simulink model "path_tracker_demo"  (R2019b)
settings: Solver=FixedStepDiscrete  StartTime=0.0  StopTime=40  FixedStep=0.01  RelTol=1e-3  EnableMultiTasking=on
undefined symbols (not defined in the file or in its folder): DiscIntNeverNeededParam, path_data_D
libraries: simulink x3
Description:
  | Counter Implemented in a C++ S-function
settings Model: ExtModeTrigMode=oneshot  ExtModeArmWhenConnect=off  ExtModeAutoUpdateStatusClock=off  Creator=The MathWorks, Inc.  LastModifiedBy=chr
settings DataIOCC: SaveFormat=Array
settings OptimizationCC: BlockReduction=off  BooleanDataType=off  ExpressionDepthLimit=2147483647  InitFltsAndDblsToZero=on  LifeSpan=inf
settings DebuggingCC: SaveWithParameterizedLinksMsg=none  SignalResolutionControl=TryResolveAllWithWarning  MultiTaskDSMMsg=warning  MultiTaskCondExecSysMsg=none  FcnCallInpInsideContextMsg=warning  StateNameClashWarn=warning  SFUnexpectedBacktrackingDiag=warning  SFNoUnconditionalDefaultTransitionDiag=warning  SFExecutionAtInitializationDiag=none  ArithmeticOperatorsInVariantConditions=warning
settings HardwareCC: ProdBitPerPointer=32  ProdBitPerSizeT=32  ProdBitPerPtrDiffT=32  ProdLargestAtomicFloat=None  ProdIntDivRoundTo=Undefined  ProdEndianess=Unspecified  ProdWordSize=32  ProdHWDeviceType=32-bit Generic
settings ModelReferenceCC: PropagateSignalLabelsOutOfModel=off
settings SFSimCC: SimUseLocalCustomCode=off  CustomCodeUndefinedFunction=UseInterfaceOnly
settings RTWCC: Description=Generic Real-Time Target  RetainRTWFile=on  RTWUseLocalCustomCode=off
settings CodeAppCC: StateflowObjectComments=on
settings GRTTargetCC: TargetFcnLib=ansi_tfl_tmw.mat  TargetLangStandard=C89/C90 (ANSI)  GeneratePreprocessorConditionals=Disable all  CombineOutputUpdateFcns=off  GRTInterface=on
settings ConfigComp: CovMetricSettings=dw  CovHtmlReporting=on  CovSaveCumulativeToWorkspaceVar=on  CovSaveSingleToWorkspaceVar=on  CovExternalEMLEnable=off

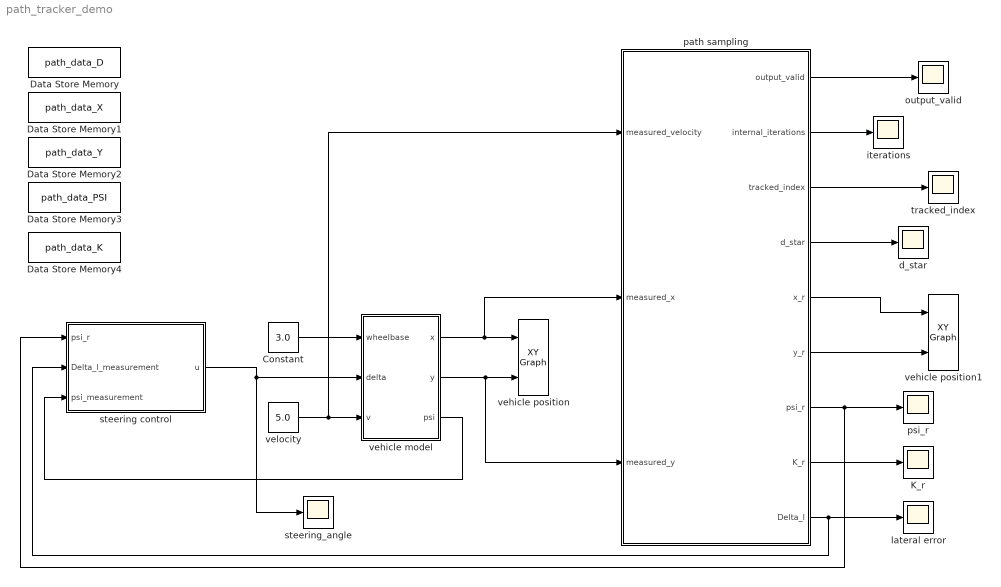
== system path_tracker_demo ==
  Constant : Constant  Value=3.0
  Data Store Memory : DataStoreMemory  DataStoreName=path_data_D  ReadBeforeWriteMsg=warning  WriteAfterWriteMsg=warning  WriteAfterReadMsg=warning  InitialValue=path_data.D  ShowAdditionalParam=off
  Data Store Memory1 : DataStoreMemory  DataStoreName=path_data_X  ReadBeforeWriteMsg=warning  WriteAfterWriteMsg=warning  WriteAfterReadMsg=warning  InitialValue=path_data.X  ShowAdditionalParam=off
  Data Store Memory2 : DataStoreMemory  DataStoreName=path_data_Y  ReadBeforeWriteMsg=warning  WriteAfterWriteMsg=warning  WriteAfterReadMsg=warning  InitialValue=path_data.Y  ShowAdditionalParam=off
  Data Store Memory3 : DataStoreMemory  DataStoreName=path_data_PSI  ReadBeforeWriteMsg=warning  WriteAfterWriteMsg=warning  WriteAfterReadMsg=warning  InitialValue=path_data.PSI  ShowAdditionalParam=off
  Data Store Memory4 : DataStoreMemory  DataStoreName=path_data_K  ReadBeforeWriteMsg=warning  WriteAfterWriteMsg=warning  WriteAfterReadMsg=warning  InitialValue=path_data.K  ShowAdditionalParam=off
  K_r : Scope
  d_star : Scope
  iterations : Scope
  lateral error : Scope
  output_valid : Scope
  path sampling : Subsystem
  psi_r : Scope
  steering control : Subsystem
  steering_angle : Scope
  tracked_index : Scope
  vehicle position : simulink/Sinks/XY Graph  xmin=-40  xmax=40  ymin=-40  ymax=40  st=-1
  vehicle position1 : simulink/Sinks/XY Graph  xmin=-40  xmax=40  ymin=-40  ymax=40  st=-1
  vehicle model : Subsystem
  velocity : Constant  Value=5.0
  wires:
  path sampling/1(output_valid) -> output_valid/1
  path sampling/2(internal_iterations) -> iterations/1
  path sampling/7(psi_r) -> steering control/1(psi_r), psi_r/1
  path sampling/8(K_r) -> K_r/1
  path sampling/3(tracked_index) -> tracked_index/1
  Constant/1 -> vehicle model/1(wheelbase)
  velocity/1 -> path sampling/1(measured_velocity), vehicle model/3(v)
  vehicle model/1(x) -> vehicle position/1, path sampling/2(measured_x)
  vehicle model/2(y) -> vehicle position/2, path sampling/3(measured_y)
  path sampling/5(x_r) -> vehicle position1/1
  path sampling/6(y_r) -> vehicle position1/2
  path sampling/9(Delta_l) -> steering control/2(Delta_l_measurement), lateral error/1
  path sampling/4(d_star) -> d_star/1
  steering control/1(u) -> steering_angle/1, vehicle model/2(delta)
  vehicle model/3(psi) -> steering control/3(psi_measurement)

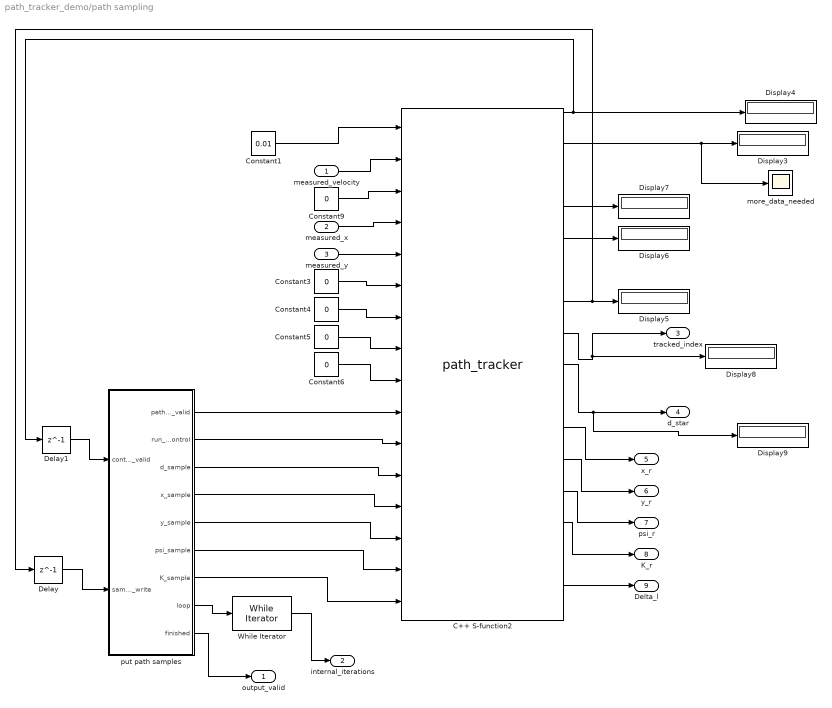
== system path_tracker_demo/path sampling ==
  measured_velocity : Inport
  measured_x : Inport  Port=2
  measured_y : Inport  Port=3
  C++ S-function2 : S-Function  FunctionName=path_tracker  Parameters=-1  SFunctionDeploymentMode=off  EnableBusSupport=off
      mask Display:
      | % copy and paste these commands into the field 'icon drawing commands' of the block mask:
      | % right-click on block -> 'Mask' -> 'Edit Mask' -> 'Mask Editor' -> 'Icons & Ports'
      | 
      | port_label('input', 1, 'Ts')
      | port_label('input', 2, 'velocity_')
      | port_label('input', 3, 'velocity_dot')
      | port_label('input', 4, 'x')
      | port_label('input', 5, 'y')
      | port_label('input', 6, 'x_dot')
      | port_label('input', 7, 'y_dot')
      | port_label('input', 8, 'Delta_u')
      | port_label('input', 9, 'Delta_u_dot')
      | port_label('input', 10, 'async_input_data_valid')
      | port_label('input', 11, 'input_sample_valid')
      | port_label('input', 12, 'd_sample')
      | port_label('input', 13, 'x_sample')
      | port_label('input', 14, 'y_sample')
      | port_label('input', 15, 'psi_sample')
      | port_label('input', 16, 'K_sample')
      | port_label('output', 1, 'output_valid')
      | port_label('output', 2, 'need_more_path_input_data')
      | port_label('output', 3, 'distance_at_the_end_of_horizon')
      | port_label('output', 4, 'distance_ahead')
      | port_label('output', 5, 'head_index')
      | port_label('output', 6, 'read_position')
      | port_label('output', 7, 'elements_free_to_write')
      | port_label('output', 8, 'tracked_index')
      | port_label('output', 9, 'd_star')
      | port_label('output', 10, 'v_star')
      | port_label('output', 11, 'x_r')
      | port_label('output', 12, 'y_r')
      | port_label('output', 13, 'psi_r')
      | port_label('output', 14, 'K_r')
      | port_label('output', 15, 'psi_r_dot')
      | port_label('output', 16, 'Delta_l')
      | port_label('output', 17, 'Delta_l_dot')
  Constant1 : Constant  Value=0.01
  Constant{3..6,9} (5 alike) : Constant  Value=0
  Delay : Delay  DelayLength=1  InitialCondition=0
  Delay1 : Delay  DelayLength=1  InitialCondition=0
  Display{3..9} (7 alike) : Display
  While Iterator : WhileIterator  MaxIters=1000  WhileBlockType=do-while  ShowIterationPort=on
  more_data_needed : Scope
  put path samples : Subsystem
  output_valid : Outport
  internal_iterations : Outport  Port=2
  tracked_index : Outport  Port=3
  d_star : Outport  Port=4
  x_r : Outport  Port=5
  y_r : Outport  Port=6
  psi_r : Outport  Port=7
  K_r : Outport  Port=8
  Delta_l : Outport  Port=9
  wires:
  C++ S-function2/5 -> Display6/1
  Constant4/1 -> C++ S-function2/7
  measured_y/1 -> C++ S-function2/5
  Constant6/1 -> C++ S-function2/9
  C++ S-function2/8 -> Display8/1, tracked_index/1
  Constant3/1 -> C++ S-function2/6
  measured_velocity/1 -> C++ S-function2/2
  Constant1/1 -> C++ S-function2/1
  C++ S-function2/2 -> more_data_needed/1, Display3/1
  C++ S-function2/9 -> Display9/1, d_star/1
  Constant5/1 -> C++ S-function2/8
  C++ S-function2/7 -> Display5/1, Delay/1
  Constant9/1 -> C++ S-function2/3
  C++ S-function2/1 -> Display4/1, Delay1/1
  measured_x/1 -> C++ S-function2/4
  C++ S-function2/4 -> Display7/1
  While Iterator/1 -> internal_iterations/1
  put path samples/1(path_sample_valid) -> C++ S-function2/10
  put path samples/2(run_control) -> C++ S-function2/11
  put path samples/3(d_sample) -> C++ S-function2/12
  put path samples/4(x_sample) -> C++ S-function2/13
  put path samples/5(y_sample) -> C++ S-function2/14
  put path samples/6(psi_sample) -> C++ S-function2/15
  put path samples/7(K_sample) -> C++ S-function2/16
  put path samples/8(loop) -> While Iterator/1
  put path samples/9(finished) -> output_valid/1
  Delay/1 -> put path samples/2(samples_free_to_write)
  Delay1/1 -> put path samples/1(control_output_valid)
  C++ S-function2/14 -> K_r/1
  C++ S-function2/13 -> psi_r/1
  C++ S-function2/12 -> y_r/1
  C++ S-function2/11 -> x_r/1
  C++ S-function2/16 -> Delta_l/1

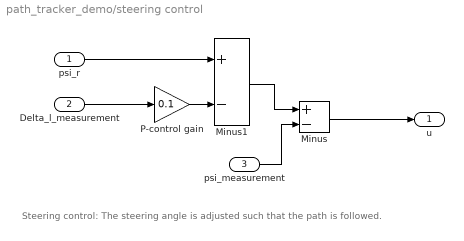
== system path_tracker_demo/steering control ==
  note: Steering control: The steering angle is adjusted such that the path is followed.
  psi_r : Inport
  Delta_l_measurement : Inport  Port=2
  psi_measurement : Inport  Port=3
  Minus : Sum  Inputs=+-
  Minus1 : Sum  Inputs=+-
  P-control gain : Gain  Gain=0.1
  u : Outport
  wires:
  psi_r/1 -> Minus1/1
  Minus/1 -> u/1
  P-control gain/1 -> Minus1/2
  psi_measurement/1 -> Minus/2
  Delta_l_measurement/1 -> P-control gain/1
  Minus1/1 -> Minus/1

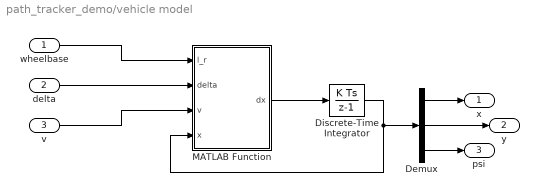
== system path_tracker_demo/vehicle model ==
  wheelbase : Inport
  delta : Inport  Port=2
  v : Inport  Port=3
  Demux : Demux  Outputs=[1;1;1]
  Discrete-Time Integrator : DiscreteIntegrator  InitialCondition=[0; 0; 0]  SampleTime=-1  ICPrevOutput=DiscIntNeverNeededParam  ICPrevScaledInput=DiscIntNeverNeededParam
  MATLAB Function : MATLAB Function  TreatAsAtomicUnit=on
  x : Outport
  y : Outport  Port=2
  psi : Outport  Port=3
  wires:
  Demux/1 -> x/1
  Demux/3 -> psi/1
  Demux/2 -> y/1
  wheelbase/1 -> MATLAB Function/1(l_r)
  delta/1 -> MATLAB Function/2(delta)
  MATLAB Function/1(dx) -> Discrete-Time Integrator/1
  v/1 -> MATLAB Function/3(v)
  Discrete-Time Integrator/1 -> Demux/1, MATLAB Function/4(x)

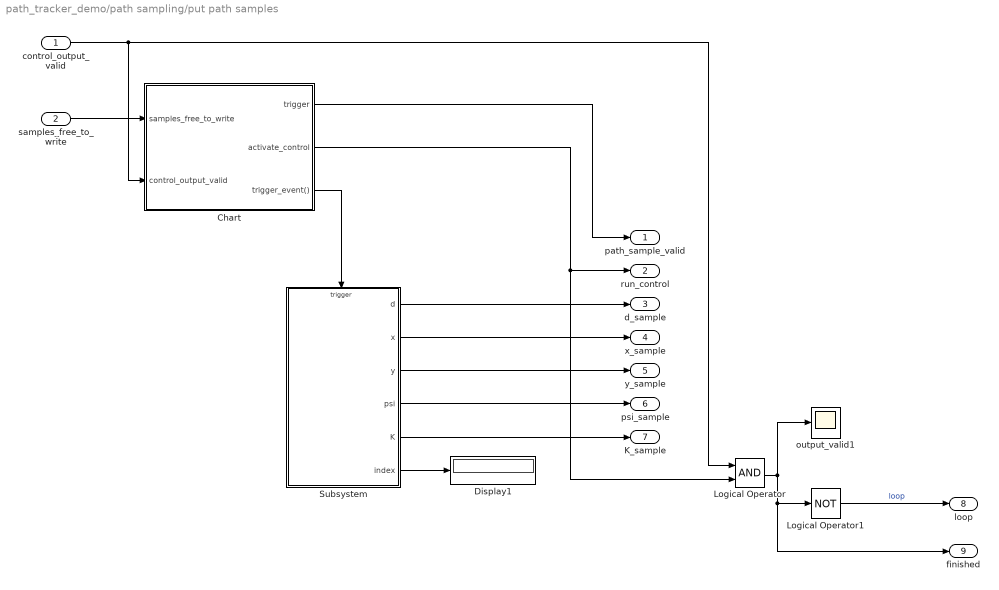
== system path_tracker_demo/path sampling/put path samples ==
  control_output_valid : Inport
  samples_free_to_write : Inport  Port=2
  Chart : Stateflow chart  BlockKeywords=__PRM__SERIALIZED__DATA__:Stateflow Chart,Stateflow Diagram  TreatAsAtomicUnit=on
  Display1 : Display
  Logical Operator : Logic  AllPortsSameDT=off  OutDataTypeStr=boolean
  Logical Operator1 : Logic  Operator=NOT  AllPortsSameDT=off  OutDataTypeStr=boolean
  Subsystem : Subsystem
  output_valid1 : Scope
  path_sample_valid : Outport
  run_control : Outport  Port=2
  d_sample : Outport  Port=3
  x_sample : Outport  Port=4
  y_sample : Outport  Port=5
  psi_sample : Outport  Port=6
  K_sample : Outport  Port=7
  loop : Outport  Port=8
  finished : Outport  Port=9
  wires:
  Logical Operator1/1 -> loop/1  "loop"
  Chart/1(trigger) -> path_sample_valid/1
  Subsystem/1(d) -> d_sample/1
  Subsystem/4(psi) -> psi_sample/1
  Subsystem/2(x) -> x_sample/1
  Subsystem/3(y) -> y_sample/1
  Subsystem/5(K) -> K_sample/1
  Logical Operator/1 -> finished/1, Logical Operator1/1, output_valid1/1
  control_output_valid/1 -> Chart/2(control_output_valid), Logical Operator/1
  Chart/2(activate_control) -> run_control/1, Logical Operator/2
  Subsystem/6(index) -> Display1/1
  Chart/3(trigger_event()) -> Subsystem/Trigger
  samples_free_to_write/1 -> Chart/1(samples_free_to_write)

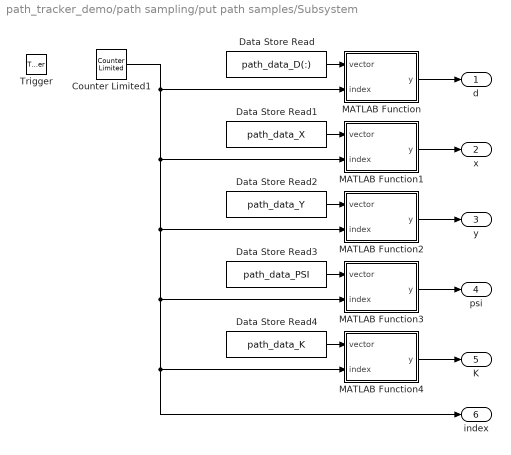
== system path_tracker_demo/path sampling/put path samples/Subsystem ==
  Trigger : TriggerPort  TriggerType=function-call  VariantControl=Variant  PortDimensions=1
  Counter Limited1 : simulink/Sources/Counter Limited  uplimit=path_data.N - 1  tsamp=-1
  Data Store Read : DataStoreRead  DataStoreName=path_data_D  DataStoreElements=path_data_D(:)
  Data Store Read1 : DataStoreRead  DataStoreName=path_data_X
  Data Store Read2 : DataStoreRead  DataStoreName=path_data_Y
  Data Store Read3 : DataStoreRead  DataStoreName=path_data_PSI
  Data Store Read4 : DataStoreRead  DataStoreName=path_data_K
  MATLAB Function : MATLAB Function  TreatAsAtomicUnit=on
  MATLAB Function1 : MATLAB Function  TreatAsAtomicUnit=on
  MATLAB Function2 : MATLAB Function  TreatAsAtomicUnit=on
  MATLAB Function3 : MATLAB Function  TreatAsAtomicUnit=on
  MATLAB Function4 : MATLAB Function  TreatAsAtomicUnit=on
  d : Outport
  x : Outport  Port=2
  y : Outport  Port=3
  psi : Outport  Port=4
  K : Outport  Port=5
  index : Outport  Port=6
  wires:
  Data Store Read/1 -> MATLAB Function/1(vector)
  MATLAB Function/1(y) -> d/1
  MATLAB Function1/1(y) -> x/1
  Data Store Read1/1 -> MATLAB Function1/1(vector)
  MATLAB Function2/1(y) -> y/1
  Data Store Read2/1 -> MATLAB Function2/1(vector)
  MATLAB Function3/1(y) -> psi/1
  Data Store Read3/1 -> MATLAB Function3/1(vector)
  Counter Limited1/1 -> index/1, MATLAB Function4/2(index), MATLAB Function3/2(index), MATLAB Function2/2(index), MATLAB Function1/2(index), MATLAB Function/2(index)
  MATLAB Function4/1(y) -> K/1
  Data Store Read4/1 -> MATLAB Function4/1(vector)

== matlab function path_tracker_demo/path sampling/put path samples/Subsystem/MATLAB Function ==
  data: vector input; y output; index input
function y = fcn(vector, index)

y = vector(index+1);

== matlab function path_tracker_demo/path sampling/put path samples/Subsystem/MATLAB Function1 ==
  data: vector input; y output; index input
function y = fcn(vector, index)

y = vector(index+1);

== stateflow chart path_tracker_demo/path sampling/put path samples/Chart ==
  state init
    trigger=false;
    activate_control=false;
  state fill_buffer
    bind: trigger_event;
    en, du: trigger_event;
    trigger=true;
    activate_control=false;
  state buffer_filled
    trigger=false;
    activate_control=true;
  (default) -> init
  init -> fill_buffer : after(2, tick)
  buffer_filled -> fill_buffer [order 2] : [~control_output_valid]
  fill_buffer -> buffer_filled [order 2] : [samples_free_to_write <= 1]
  buffer_filled -> fill_buffer [order 1] : after(100,tick)
  fill_buffer -> buffer_filled [order 1] : after(50, tick)
  data: trigger output boolean; activate_control output boolean; samples_free_to_write input size=1; control_output_valid input size=1
  events: trigger_event output FUNCTION_CALL_EVENT

== matlab function path_tracker_demo/path sampling/put path samples/Subsystem/MATLAB Function2 ==
  data: vector input; y output; index input
function y = fcn(vector, index)

y = vector(index+1);

== matlab function path_tracker_demo/path sampling/put path samples/Subsystem/MATLAB Function3 ==
  data: vector input; y output; index input
function y = fcn(vector, index)

y = vector(index+1);

== matlab function path_tracker_demo/path sampling/put path samples/Subsystem/MATLAB Function4 ==
  data: vector input; y output; index input
function y = fcn(vector, index)

y = vector(index+1);

== matlab function path_tracker_demo/vehicle model/MATLAB Function ==
  data: l_r input; delta input; v input; dx output; x input
function dx = fcn(l_r, delta, v, x)

dx = [
    v * cos(delta + x(3));
    v * sin(delta + x(3));
    v / l_r * sin(delta)
];
